simulink model "untitled1"  (R2024a)
settings: Solver=FixedStepDiscrete  StartTime=0.0  StopTime=10.0  RelTol=1e-3
model workspace (MAT data in the model file):
  firstWarning = 1
  originalScenarioChecksum = '2812A957B9DD70FFB07C7DC8FD622341'
undefined symbols (not defined in the file): driving, matlabshared, rcsSignature
libraries: drivingscenarioandsensors x6, radarlib x2, lidarlib x1, sensorinslib x1
(part 1 of 2)
settings Model: Creator=44ays  LastModifiedBy=44ays

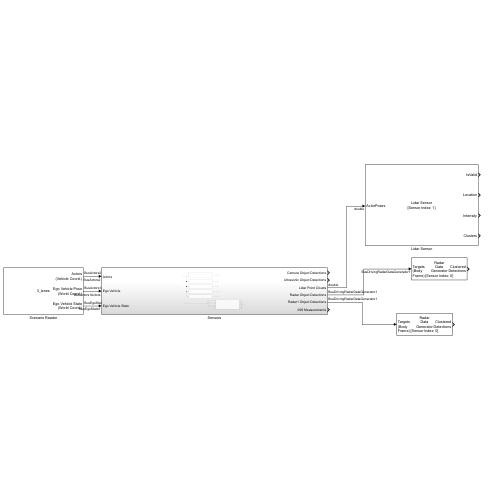
[thumbnail: Simulink's stored preview of the top-level diagram]
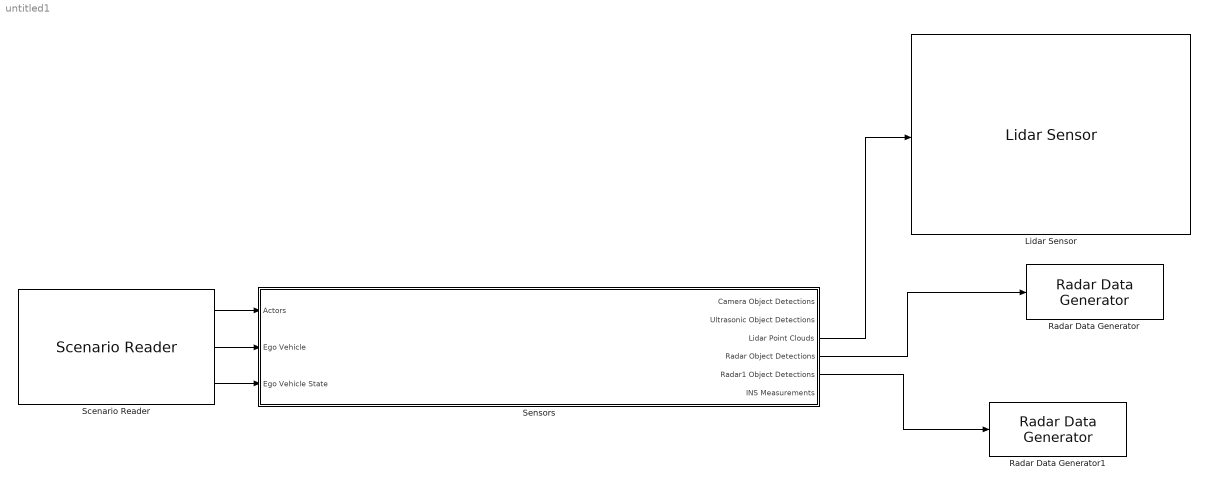
== system untitled1 ==
  Lidar Sensor : lidarlib/Lidar Sensor  SensorIndex=1  UpdateRate=0.1  Model=Custom  SensorPosition=[1.5 0 1.6]  SensorOrientation=[0 0 0]  ActorProfilesVariableName=actor_profiles  HostID=1  MaxRange=120  AzimuthLimits=[-180 180]  AzimuthResolution=0.16  UseCustomElevationAngles=off  ElevationAngles=[-25 -15.6 -11.3 -8.8:0.9:-4 -4:0.32:1.6 3.3 4.6 7 10.3 15]  ElevationLimits=[-20 20]  ElevationResolution=1.25  HasNoise=on  RangeAccuracy=0.002  FogVisibility=1000  Rainrate=0  HasMotionDistortion=off  FiringTimes=[]  OutputIntensity=on  OutputClusters=on
  Radar Data Generator : radarlib/Radar Data Generator  SensorIndex=0  UpdateRate=10  MountingLocation=[ 3.4, 0, 0.2 ]  MountingAngles=[0 0 0]  ScanMode=No scanning  HasElevation=off  HasRangeRate=on  HasNoise=on  HasFalseAlarms=on  HasOcclusion=on  HasGhosts=off  MaxNumReportsSource=Property  MaxNumReports=50  TargetReportFormat=Clustered detections  DetectionCoordinates=Body  TrackCoordinates=Body  TimeInputSource=Auto  HasINS=off  BusNameSource=Auto  BusName=BusRadarDataGenerator  HasConfigurationOutput=off  BusName2Source=Auto  BusName2=BusRadarDataGeneratorConfig  AzimuthResolution=4  ElevationResolution=5  RangeResolution=2.5  RangeRateResolution=0.5  AzimuthBiasFraction=0.1  ElevationBiasFraction=0.1  RangeBiasFraction=0.05  RangeRateBiasFraction=0.05  FieldOfView=[ 20, 5 ]  RangeLimits=[ 0, 150 ]  RangeRateLimits=[ -100, 100 ]  DetectionProbability=0.9  FalseAlarmRate=1e-06  ReferenceRange=100  ReferenceRCS=0  CenterFrequency=77e9  FilterInitializationFcn=initcvekf  ConfirmationThreshold=[2 3]  DeletionThreshold=[5 5]  InitialSeedSource=Repeatable  InitialSeed=0  UsedSeed=matlabshared.tracking.internal.SimulinkUtilities.seedManager(gcb)  ProfilesSource=From Scenario Reader block  ProfilesParameters=matlabshared.tracking.internal.PlatformProfilesRadarParameters  ProfilesExpression=struct('ClassID',0,'Dimensions',struct('Length',0,'Width',0,'Height',0,'OriginOffset',[0 0 0]),'Signatures',{{rcsSignature}})
  Radar Data Generator1 : radarlib/Radar Data Generator  SensorIndex=0  UpdateRate=10  MountingLocation=[ 3.4, 0, 0.2 ]  MountingAngles=[0 0 0]  ScanMode=No scanning  HasElevation=off  HasRangeRate=on  HasNoise=on  HasFalseAlarms=on  HasOcclusion=on  HasGhosts=off  MaxNumReportsSource=Property  MaxNumReports=50  TargetReportFormat=Clustered detections  DetectionCoordinates=Body  TrackCoordinates=Body  TimeInputSource=Auto  HasINS=off  BusNameSource=Auto  BusName=BusRadarDataGenerator  HasConfigurationOutput=off  BusName2Source=Auto  BusName2=BusRadarDataGeneratorConfig  AzimuthResolution=4  ElevationResolution=5  RangeResolution=2.5  RangeRateResolution=0.5  AzimuthBiasFraction=0.1  ElevationBiasFraction=0.1  RangeBiasFraction=0.05  RangeRateBiasFraction=0.05  FieldOfView=[ 20, 5 ]  RangeLimits=[ 0, 150 ]  RangeRateLimits=[ -100, 100 ]  DetectionProbability=0.9  FalseAlarmRate=1e-06  ReferenceRange=100  ReferenceRCS=0  CenterFrequency=77e9  FilterInitializationFcn=initcvekf  ConfirmationThreshold=[2 3]  DeletionThreshold=[5 5]  InitialSeedSource=Repeatable  InitialSeed=0  UsedSeed=matlabshared.tracking.internal.SimulinkUtilities.seedManager(gcb)  ProfilesSource=From Scenario Reader block  ProfilesParameters=matlabshared.tracking.internal.PlatformProfilesRadarParameters  ProfilesExpression=struct('ClassID',0,'Dimensions',struct('Length',0,'Width',0,'Height',0,'OriginOffset',[0 0 0]),'Signatures',{{rcsSignature}})
  Scenario Reader : drivingscenarioandsensors/Scenario Reader  ScenarioSource=From file  ScenarioFileName=D:\Belgeler\Matlab Uygulamalar\6-Driving Scenario Designer\3_lanes\3_lanes.mat  ScenarioVariableName=scenario  OutputCoordinateSystem=Vehicle coordinates  EgoVehicleSource=Scenario  EgoVehicleActorID=1  OrientVehiclesOnRoad=off  OutputEgoVehiclePose=on  OutputEgoVehicleState=on  SampleTime=0.1  LaneBoundaryOutput=None  LaneBoundaryDistance=0:0.5:9.5  LaneBoundaryLocation=Center of lane markings  BusNameSource=Auto  BusName=BusActors  BusNumActorsSource=Scenario  BusNumActors=100  BusName2Source=Auto  BusName2=BusLaneBoundaries  BusNumLaneBoundariesSource=Scenario  BusNumLaneBoundaries=10  BusName3Source=Auto  BusName3=BusEgoActor  BusName4Source=Auto  BusName4=BusEgoState  ShowCoordinateLabels=on  SimulateUsing=Interpreted execution
  Sensors : Subsystem
  wires:
  Scenario Reader/2 -> Sensors/2(Ego Vehicle)
  Scenario Reader/1 -> Sensors/1(Actors)
  Scenario Reader/3 -> Sensors/3(Ego Vehicle State)
  Sensors/3(Lidar Point Clouds) -> Lidar Sensor/1
  Sensors/4(Radar Object Detections) -> Radar Data Generator/1
  Sensors/5(Radar1 Object Detections) -> Radar Data Generator1/1
